simulink model "TST_OilT_VD"  (R2016b)
settings: Solver=FixedStepDiscrete  StartTime=0.0  StopTime=simTime  FixedStep=sampleTime  RelTol=1e-3
values from neighbouring files (symbols this model uses):
  testCase = 1    [initTST_OilT_VD_001.m]    (also in initTST_OilT_VD_002.m = 2)
libraries: UnitTest_Lib x8, simulink x3
settings Model: Creator=liangyunbo  LastModifiedBy=liangyunbo
settings DebuggingCC: SignalRangeChecking=error

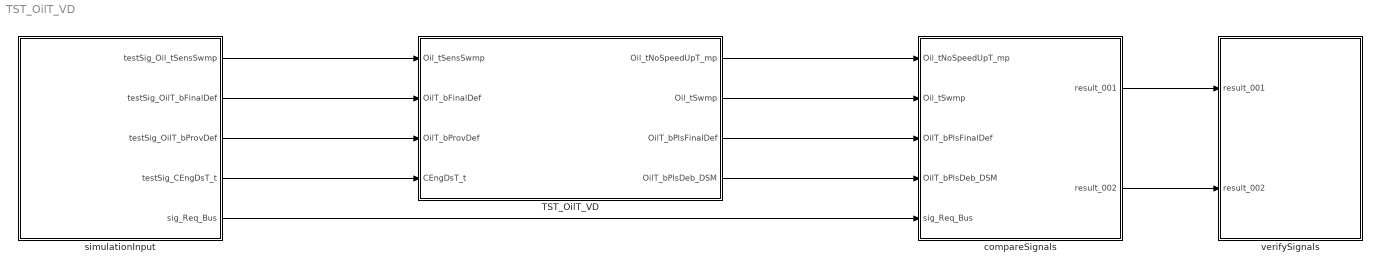
== system TST_OilT_VD ==
  TST_OilT_VD : Subsystem
  compareSignals : Subsystem
  simulationInput : Subsystem
  verifySignals : Subsystem
  wires:
  simulationInput/1(testSig_Oil_tSensSwmp) -> TST_OilT_VD/1(Oil_tSensSwmp)
  simulationInput/2(testSig_OilT_bFinalDef) -> TST_OilT_VD/2(OilT_bFinalDef)
  simulationInput/3(testSig_OilT_bProvDef) -> TST_OilT_VD/3(OilT_bProvDef)
  simulationInput/4(testSig_CEngDsT_t) -> TST_OilT_VD/4(CEngDsT_t)
  TST_OilT_VD/1(Oil_tNoSpeedUpT_mp) -> compareSignals/1(Oil_tNoSpeedUpT_mp)
  TST_OilT_VD/2(Oil_tSwmp) -> compareSignals/2(Oil_tSwmp)
  TST_OilT_VD/3(OilT_bPlsFinalDef) -> compareSignals/3(OilT_bPlsFinalDef)
  TST_OilT_VD/4(OilT_bPlsDeb_DSM) -> compareSignals/4(OilT_bPlsDeb_DSM)
  simulationInput/5(sig_Req_Bus) -> compareSignals/5(sig_Req_Bus)
  compareSignals/1(result_001) -> verifySignals/1(result_001)
  compareSignals/2(result_002) -> verifySignals/2(result_002)

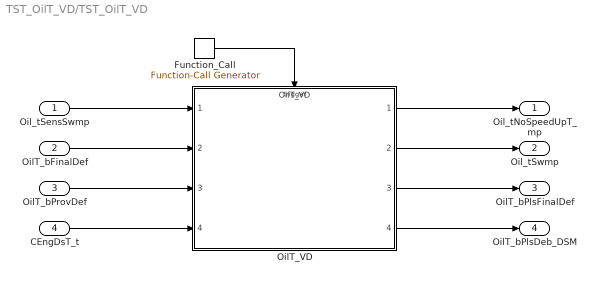
== system TST_OilT_VD/TST_OilT_VD ==
  Oil_tSensSwmp : Inport
  OilT_bFinalDef : Inport  Port=2
  OilT_bProvDef : Inport  Port=3
  CEngDsT_t : Inport  Port=4
  Function_Call : simulink/Ports & Subsystems/Function-Call Generator  sample_time=sampleTime  numberOfIterations=1
  OilT_VD : ModelReference  ModelNameDialog=OilT_VD  SimulationMode=Normal  ModelReferenceVersion=1.9  TriggerPortName=function  TriggerPortTriggerType=function-call  TriggerPortStatesWhenEnabling=held
  Oil_tNoSpeedUpT_mp : Outport
  Oil_tSwmp : Outport  Port=2
  OilT_bPlsFinalDef : Outport  Port=3
  OilT_bPlsDeb_DSM : Outport  Port=4
  wires:
  Function_Call/1 -> OilT_VD/Trigger
  Oil_tSensSwmp/1 -> OilT_VD/1
  OilT_bFinalDef/1 -> OilT_VD/2
  OilT_bProvDef/1 -> OilT_VD/3
  CEngDsT_t/1 -> OilT_VD/4
  OilT_VD/1 -> Oil_tNoSpeedUpT_mp/1
  OilT_VD/2 -> Oil_tSwmp/1
  OilT_VD/3 -> OilT_bPlsFinalDef/1
  OilT_VD/4 -> OilT_bPlsDeb_DSM/1

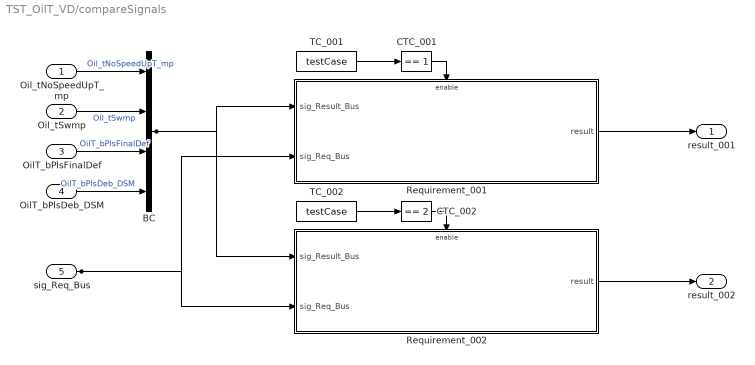
== system TST_OilT_VD/compareSignals ==
  Oil_tNoSpeedUpT_mp : Inport
  Oil_tSwmp : Inport  Port=2
  OilT_bPlsFinalDef : Inport  Port=3
  OilT_bPlsDeb_DSM : Inport  Port=4
  sig_Req_Bus : Inport  Port=5
  BC : BusCreator  Inputs=4
  CTC_001 : simulink/Logic and Bit Operations/Compare To Constant  relop===  const=1  OutDataTypeStr=boolean
  CTC_002 : simulink/Logic and Bit Operations/Compare To Constant  relop===  const=2  OutDataTypeStr=boolean
  Requirement_001 : Subsystem
  Requirement_002 : Subsystem
  TC_001 : Constant  Value=testCase
  TC_002 : Constant  Value=testCase
  result_001 : Outport
  result_002 : Outport  Port=2
  wires:
  Oil_tNoSpeedUpT_mp/1 -> BC/1  "Oil_tNoSpeedUpT_mp"
  Oil_tSwmp/1 -> BC/2  "Oil_tSwmp"
  OilT_bPlsFinalDef/1 -> BC/3  "OilT_bPlsFinalDef"
  OilT_bPlsDeb_DSM/1 -> BC/4  "OilT_bPlsDeb_DSM"
  TC_001/1 -> CTC_001/1
  CTC_001/1 -> Requirement_001/Enable
  sig_Req_Bus/1 -> Requirement_001/2(sig_Req_Bus), Requirement_002/2(sig_Req_Bus)
  BC/1 -> Requirement_001/1(sig_Result_Bus), Requirement_002/1(sig_Result_Bus)
  Requirement_001/1(result) -> result_001/1
  TC_002/1 -> CTC_002/1
  CTC_002/1 -> Requirement_002/Enable
  Requirement_002/1(result) -> result_002/1

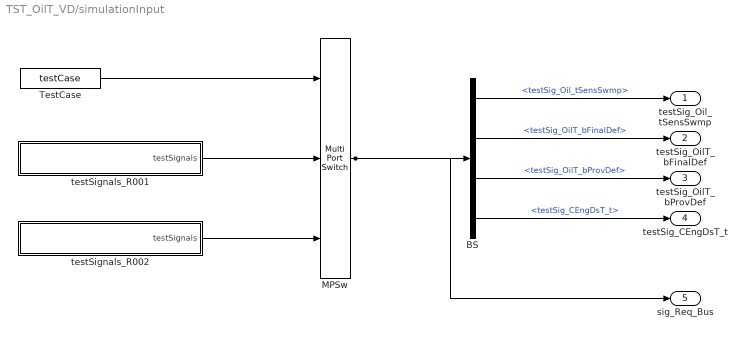
== system TST_OilT_VD/simulationInput ==
  BS : BusSelector  OutputSignals=testSig_Oil_tSensSwmp,testSig_OilT_bFinalDef,testSig_OilT_bProvDef,testSig_CEngDsT_t
  MPSw : MultiPortSwitch  Inputs=2  SaturateOnIntegerOverflow=on  InputSameDT=on
  TestCase : Constant  Value=testCase
  testSignals_R001 : Subsystem
  testSignals_R002 : Subsystem
  testSig_Oil_tSensSwmp : Outport
  testSig_OilT_bFinalDef : Outport  Port=2
  testSig_OilT_bProvDef : Outport  Port=3
  testSig_CEngDsT_t : Outport  Port=4
  sig_Req_Bus : Outport  Port=5
  wires:
  BS/1 -> testSig_Oil_tSensSwmp/1  "<testSig_Oil_tSensSwmp>"
  BS/2 -> testSig_OilT_bFinalDef/1  "<testSig_OilT_bFinalDef>"
  BS/3 -> testSig_OilT_bProvDef/1  "<testSig_OilT_bProvDef>"
  BS/4 -> testSig_CEngDsT_t/1  "<testSig_CEngDsT_t>"
  MPSw/1 -> BS/1, sig_Req_Bus/1
  TestCase/1 -> MPSw/1
  testSignals_R001/1(testSignals) -> MPSw/2
  testSignals_R002/1(testSignals) -> MPSw/3

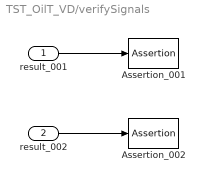
== system TST_OilT_VD/verifySignals ==
  result_001 : Inport
  result_002 : Inport  Port=2
  Assertion_001 : Assertion  Enabled=off
  Assertion_002 : Assertion  Enabled=off
  wires:
  result_001/1 -> Assertion_001/1
  result_002/1 -> Assertion_002/1

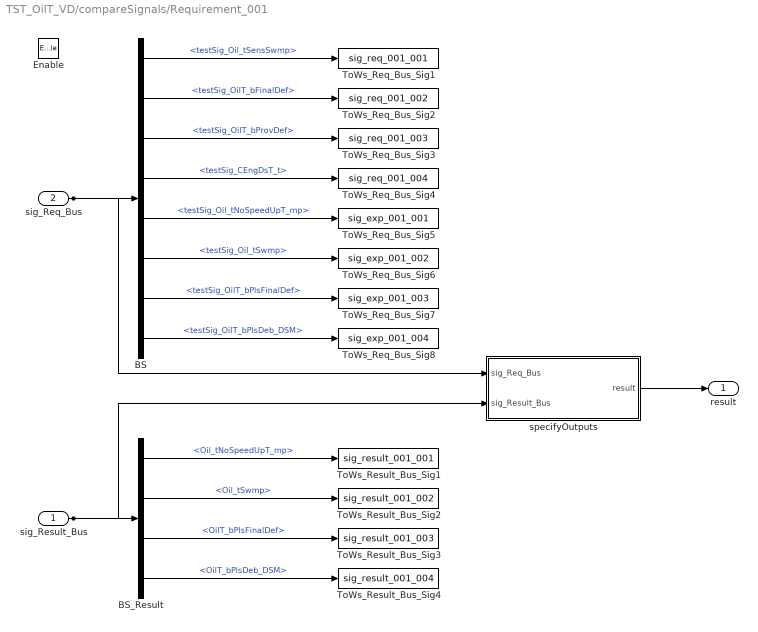
== system TST_OilT_VD/compareSignals/Requirement_001 ==
  sig_Result_Bus : Inport
  sig_Req_Bus : Inport  Port=2
  Enable : EnablePort
  BS : BusSelector  OutputSignals=testSig_Oil_tSensSwmp,testSig_OilT_bFinalDef,testSig_OilT_bProvDef,testSig_CEngDsT_t,testSig_Oil_tNoSpeedUpT_mp,testSig_Oil_tSwmp,testSig_OilT_bPlsFinalDef,testSig_OilT_bPlsDeb_DSM
  BS_Result : BusSelector  OutputSignals=Oil_tNoSpeedUpT_mp,Oil_tSwmp,OilT_bPlsFinalDef,OilT_bPlsDeb_DSM
  ToWs_Req_Bus_Sig1 : ToWorkspace  VariableName=sig_req_001_001  SaveFormat=Structure With Time
  ToWs_Req_Bus_Sig2 : ToWorkspace  VariableName=sig_req_001_002  SaveFormat=Structure With Time
  ToWs_Req_Bus_Sig3 : ToWorkspace  VariableName=sig_req_001_003  SaveFormat=Structure With Time
  ToWs_Req_Bus_Sig4 : ToWorkspace  VariableName=sig_req_001_004  SaveFormat=Structure With Time
  ToWs_Req_Bus_Sig5 : ToWorkspace  VariableName=sig_exp_001_001  SaveFormat=Structure With Time
  ToWs_Req_Bus_Sig6 : ToWorkspace  VariableName=sig_exp_001_002  SaveFormat=Structure With Time
  ToWs_Req_Bus_Sig7 : ToWorkspace  VariableName=sig_exp_001_003  SaveFormat=Structure With Time
  ToWs_Req_Bus_Sig8 : ToWorkspace  VariableName=sig_exp_001_004  SaveFormat=Structure With Time
  ToWs_Result_Bus_Sig1 : ToWorkspace  VariableName=sig_result_001_001  SaveFormat=Structure With Time
  ToWs_Result_Bus_Sig2 : ToWorkspace  VariableName=sig_result_001_002  SaveFormat=Structure With Time
  ToWs_Result_Bus_Sig3 : ToWorkspace  VariableName=sig_result_001_003  SaveFormat=Structure With Time
  ToWs_Result_Bus_Sig4 : ToWorkspace  VariableName=sig_result_001_004  SaveFormat=Structure With Time
  specifyOutputs : Subsystem
  result : Outport
  wires:
  sig_Req_Bus/1 -> BS/1, specifyOutputs/1(sig_Req_Bus)
  BS/1 -> ToWs_Req_Bus_Sig1/1  "<testSig_Oil_tSensSwmp>"
  BS/2 -> ToWs_Req_Bus_Sig2/1  "<testSig_OilT_bFinalDef>"
  BS/3 -> ToWs_Req_Bus_Sig3/1  "<testSig_OilT_bProvDef>"
  BS/4 -> ToWs_Req_Bus_Sig4/1  "<testSig_CEngDsT_t>"
  BS/5 -> ToWs_Req_Bus_Sig5/1  "<testSig_Oil_tNoSpeedUpT_mp>"
  BS/6 -> ToWs_Req_Bus_Sig6/1  "<testSig_Oil_tSwmp>"
  BS/7 -> ToWs_Req_Bus_Sig7/1  "<testSig_OilT_bPlsFinalDef>"
  BS/8 -> ToWs_Req_Bus_Sig8/1  "<testSig_OilT_bPlsDeb_DSM>"
  sig_Result_Bus/1 -> BS_Result/1, specifyOutputs/2(sig_Result_Bus)
  BS_Result/1 -> ToWs_Result_Bus_Sig1/1  "<Oil_tNoSpeedUpT_mp>"
  BS_Result/2 -> ToWs_Result_Bus_Sig2/1  "<Oil_tSwmp>"
  BS_Result/3 -> ToWs_Result_Bus_Sig3/1  "<OilT_bPlsFinalDef>"
  BS_Result/4 -> ToWs_Result_Bus_Sig4/1  "<OilT_bPlsDeb_DSM>"
  specifyOutputs/1(result) -> result/1

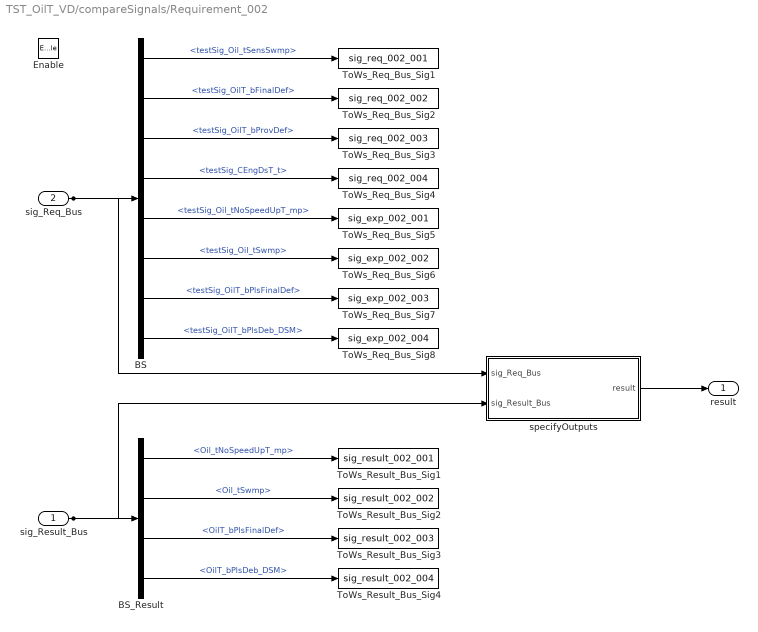
== system TST_OilT_VD/compareSignals/Requirement_002 ==
  sig_Result_Bus : Inport
  sig_Req_Bus : Inport  Port=2
  Enable : EnablePort
  BS : BusSelector  OutputSignals=testSig_Oil_tSensSwmp,testSig_OilT_bFinalDef,testSig_OilT_bProvDef,testSig_CEngDsT_t,testSig_Oil_tNoSpeedUpT_mp,testSig_Oil_tSwmp,testSig_OilT_bPlsFinalDef,testSig_OilT_bPlsDeb_DSM
  BS_Result : BusSelector  OutputSignals=Oil_tNoSpeedUpT_mp,Oil_tSwmp,OilT_bPlsFinalDef,OilT_bPlsDeb_DSM
  ToWs_Req_Bus_Sig1 : ToWorkspace  VariableName=sig_req_002_001  SaveFormat=Structure With Time
  ToWs_Req_Bus_Sig2 : ToWorkspace  VariableName=sig_req_002_002  SaveFormat=Structure With Time
  ToWs_Req_Bus_Sig3 : ToWorkspace  VariableName=sig_req_002_003  SaveFormat=Structure With Time
  ToWs_Req_Bus_Sig4 : ToWorkspace  VariableName=sig_req_002_004  SaveFormat=Structure With Time
  ToWs_Req_Bus_Sig5 : ToWorkspace  VariableName=sig_exp_002_001  SaveFormat=Structure With Time
  ToWs_Req_Bus_Sig6 : ToWorkspace  VariableName=sig_exp_002_002  SaveFormat=Structure With Time
  ToWs_Req_Bus_Sig7 : ToWorkspace  VariableName=sig_exp_002_003  SaveFormat=Structure With Time
  ToWs_Req_Bus_Sig8 : ToWorkspace  VariableName=sig_exp_002_004  SaveFormat=Structure With Time
  ToWs_Result_Bus_Sig1 : ToWorkspace  VariableName=sig_result_002_001  SaveFormat=Structure With Time
  ToWs_Result_Bus_Sig2 : ToWorkspace  VariableName=sig_result_002_002  SaveFormat=Structure With Time
  ToWs_Result_Bus_Sig3 : ToWorkspace  VariableName=sig_result_002_003  SaveFormat=Structure With Time
  ToWs_Result_Bus_Sig4 : ToWorkspace  VariableName=sig_result_002_004  SaveFormat=Structure With Time
  specifyOutputs : Subsystem
  result : Outport
  wires:
  sig_Req_Bus/1 -> BS/1, specifyOutputs/1(sig_Req_Bus)
  BS/1 -> ToWs_Req_Bus_Sig1/1  "<testSig_Oil_tSensSwmp>"
  BS/2 -> ToWs_Req_Bus_Sig2/1  "<testSig_OilT_bFinalDef>"
  BS/3 -> ToWs_Req_Bus_Sig3/1  "<testSig_OilT_bProvDef>"
  BS/4 -> ToWs_Req_Bus_Sig4/1  "<testSig_CEngDsT_t>"
  BS/5 -> ToWs_Req_Bus_Sig5/1  "<testSig_Oil_tNoSpeedUpT_mp>"
  BS/6 -> ToWs_Req_Bus_Sig6/1  "<testSig_Oil_tSwmp>"
  BS/7 -> ToWs_Req_Bus_Sig7/1  "<testSig_OilT_bPlsFinalDef>"
  BS/8 -> ToWs_Req_Bus_Sig8/1  "<testSig_OilT_bPlsDeb_DSM>"
  sig_Result_Bus/1 -> BS_Result/1, specifyOutputs/2(sig_Result_Bus)
  BS_Result/1 -> ToWs_Result_Bus_Sig1/1  "<Oil_tNoSpeedUpT_mp>"
  BS_Result/2 -> ToWs_Result_Bus_Sig2/1  "<Oil_tSwmp>"
  BS_Result/3 -> ToWs_Result_Bus_Sig3/1  "<OilT_bPlsFinalDef>"
  BS_Result/4 -> ToWs_Result_Bus_Sig4/1  "<OilT_bPlsDeb_DSM>"
  specifyOutputs/1(result) -> result/1

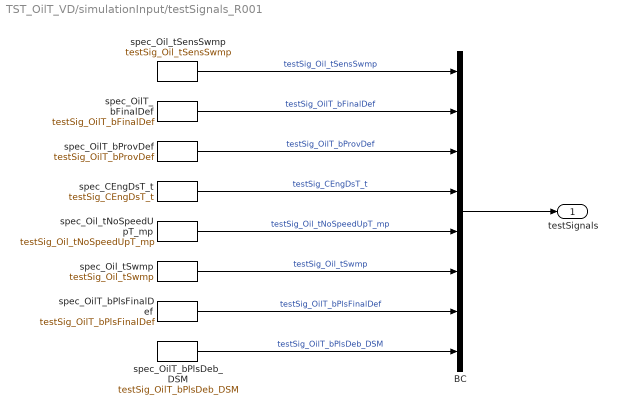
== system TST_OilT_VD/simulationInput/testSignals_R001 ==
  BC : BusCreator  Inputs=8
  spec_CEngDsT_t : FromWorkspace  VariableName=testSig_CEngDsT_t  Interpolate=off  OutputAfterFinalValue=Holding final value
  spec_OilT_bFinalDef : FromWorkspace  VariableName=testSig_OilT_bFinalDef  Interpolate=off  OutputAfterFinalValue=Holding final value
  spec_OilT_bPlsDeb_DSM : FromWorkspace  VariableName=testSig_OilT_bPlsDeb_DSM  Interpolate=off  OutputAfterFinalValue=Holding final value
  spec_OilT_bPlsFinalDef : FromWorkspace  VariableName=testSig_OilT_bPlsFinalDef  Interpolate=off  OutputAfterFinalValue=Holding final value
  spec_OilT_bProvDef : FromWorkspace  VariableName=testSig_OilT_bProvDef  Interpolate=off  OutputAfterFinalValue=Holding final value
  spec_Oil_tNoSpeedUpT_mp : FromWorkspace  VariableName=testSig_Oil_tNoSpeedUpT_mp  Interpolate=off  OutputAfterFinalValue=Holding final value
  spec_Oil_tSensSwmp : FromWorkspace  VariableName=testSig_Oil_tSensSwmp  Interpolate=off  OutputAfterFinalValue=Holding final value
  spec_Oil_tSwmp : FromWorkspace  VariableName=testSig_Oil_tSwmp  Interpolate=off  OutputAfterFinalValue=Holding final value
  testSignals : Outport
  wires:
  BC/1 -> testSignals/1
  spec_Oil_tSensSwmp/1 -> BC/1  "testSig_Oil_tSensSwmp"
  spec_OilT_bFinalDef/1 -> BC/2  "testSig_OilT_bFinalDef"
  spec_OilT_bProvDef/1 -> BC/3  "testSig_OilT_bProvDef"
  spec_CEngDsT_t/1 -> BC/4  "testSig_CEngDsT_t"
  spec_Oil_tNoSpeedUpT_mp/1 -> BC/5  "testSig_Oil_tNoSpeedUpT_mp"
  spec_Oil_tSwmp/1 -> BC/6  "testSig_Oil_tSwmp"
  spec_OilT_bPlsFinalDef/1 -> BC/7  "testSig_OilT_bPlsFinalDef"
  spec_OilT_bPlsDeb_DSM/1 -> BC/8  "testSig_OilT_bPlsDeb_DSM"

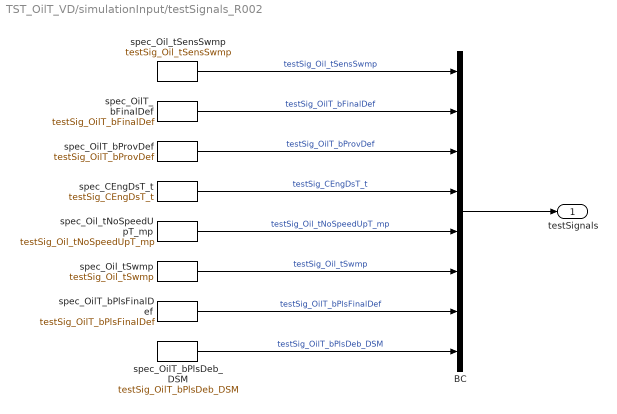
== system TST_OilT_VD/simulationInput/testSignals_R002 ==
  BC : BusCreator  Inputs=8
  spec_CEngDsT_t : FromWorkspace  VariableName=testSig_CEngDsT_t  Interpolate=off  OutputAfterFinalValue=Holding final value
  spec_OilT_bFinalDef : FromWorkspace  VariableName=testSig_OilT_bFinalDef  Interpolate=off  OutputAfterFinalValue=Holding final value
  spec_OilT_bPlsDeb_DSM : FromWorkspace  VariableName=testSig_OilT_bPlsDeb_DSM  Interpolate=off  OutputAfterFinalValue=Holding final value
  spec_OilT_bPlsFinalDef : FromWorkspace  VariableName=testSig_OilT_bPlsFinalDef  Interpolate=off  OutputAfterFinalValue=Holding final value
  spec_OilT_bProvDef : FromWorkspace  VariableName=testSig_OilT_bProvDef  Interpolate=off  OutputAfterFinalValue=Holding final value
  spec_Oil_tNoSpeedUpT_mp : FromWorkspace  VariableName=testSig_Oil_tNoSpeedUpT_mp  Interpolate=off  OutputAfterFinalValue=Holding final value
  spec_Oil_tSensSwmp : FromWorkspace  VariableName=testSig_Oil_tSensSwmp  Interpolate=off  OutputAfterFinalValue=Holding final value
  spec_Oil_tSwmp : FromWorkspace  VariableName=testSig_Oil_tSwmp  Interpolate=off  OutputAfterFinalValue=Holding final value
  testSignals : Outport
  wires:
  BC/1 -> testSignals/1
  spec_Oil_tSensSwmp/1 -> BC/1  "testSig_Oil_tSensSwmp"
  spec_OilT_bFinalDef/1 -> BC/2  "testSig_OilT_bFinalDef"
  spec_OilT_bProvDef/1 -> BC/3  "testSig_OilT_bProvDef"
  spec_CEngDsT_t/1 -> BC/4  "testSig_CEngDsT_t"
  spec_Oil_tNoSpeedUpT_mp/1 -> BC/5  "testSig_Oil_tNoSpeedUpT_mp"
  spec_Oil_tSwmp/1 -> BC/6  "testSig_Oil_tSwmp"
  spec_OilT_bPlsFinalDef/1 -> BC/7  "testSig_OilT_bPlsFinalDef"
  spec_OilT_bPlsDeb_DSM/1 -> BC/8  "testSig_OilT_bPlsDeb_DSM"

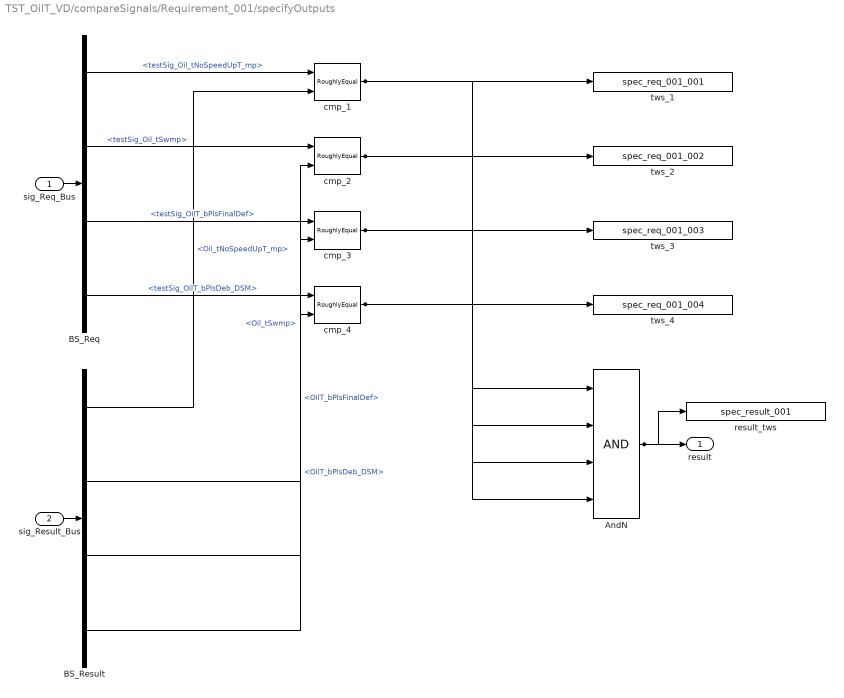
== system TST_OilT_VD/compareSignals/Requirement_001/specifyOutputs ==
  sig_Req_Bus : Inport
  sig_Result_Bus : Inport  Port=2
  AndN : Logic  Inputs=4
  BS_Req : BusSelector  OutputSignals=testSig_Oil_tNoSpeedUpT_mp,testSig_Oil_tSwmp,testSig_OilT_bPlsFinalDef,testSig_OilT_bPlsDeb_DSM
  BS_Result : BusSelector  OutputSignals=Oil_tNoSpeedUpT_mp,Oil_tSwmp,OilT_bPlsFinalDef,OilT_bPlsDeb_DSM
  cmp_{1..4} (4 alike) : UnitTest_Lib/RoughlyEqual  slope=0.1
  result_tws : ToWorkspace  VariableName=spec_result_001
  tws_1 : ToWorkspace  VariableName=spec_req_001_001
  tws_2 : ToWorkspace  VariableName=spec_req_001_002
  tws_3 : ToWorkspace  VariableName=spec_req_001_003
  tws_4 : ToWorkspace  VariableName=spec_req_001_004
  result : Outport
  wires:
  sig_Req_Bus/1 -> BS_Req/1
  sig_Result_Bus/1 -> BS_Result/1
  AndN/1 -> result/1, result_tws/1
  BS_Req/1 -> cmp_1/1  "<testSig_Oil_tNoSpeedUpT_mp>"
  BS_Result/1 -> cmp_1/2  "<Oil_tNoSpeedUpT_mp>"
  cmp_1/1 -> tws_1/1, AndN/1
  BS_Req/2 -> cmp_2/1  "<testSig_Oil_tSwmp>"
  BS_Result/2 -> cmp_2/2  "<Oil_tSwmp>"
  cmp_2/1 -> tws_2/1, AndN/2
  BS_Req/3 -> cmp_3/1  "<testSig_OilT_bPlsFinalDef>"
  BS_Result/3 -> cmp_3/2  "<OilT_bPlsFinalDef>"
  cmp_3/1 -> tws_3/1, AndN/3
  BS_Req/4 -> cmp_4/1  "<testSig_OilT_bPlsDeb_DSM>"
  BS_Result/4 -> cmp_4/2  "<OilT_bPlsDeb_DSM>"
  cmp_4/1 -> tws_4/1, AndN/4

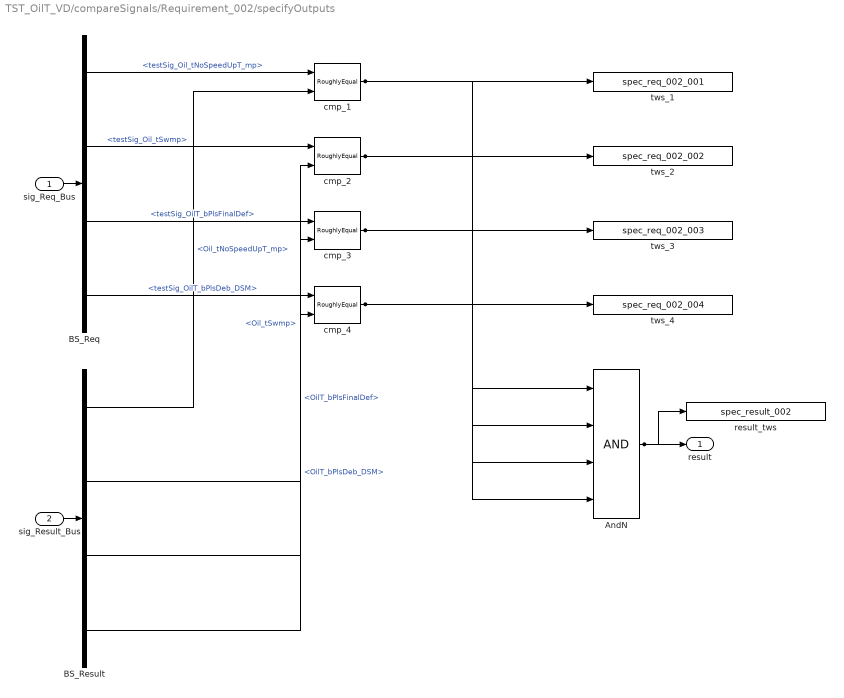
== system TST_OilT_VD/compareSignals/Requirement_002/specifyOutputs ==
  sig_Req_Bus : Inport
  sig_Result_Bus : Inport  Port=2
  AndN : Logic  Inputs=4
  BS_Req : BusSelector  OutputSignals=testSig_Oil_tNoSpeedUpT_mp,testSig_Oil_tSwmp,testSig_OilT_bPlsFinalDef,testSig_OilT_bPlsDeb_DSM
  BS_Result : BusSelector  OutputSignals=Oil_tNoSpeedUpT_mp,Oil_tSwmp,OilT_bPlsFinalDef,OilT_bPlsDeb_DSM
  cmp_{1..4} (4 alike) : UnitTest_Lib/RoughlyEqual  slope=0.1
  result_tws : ToWorkspace  VariableName=spec_result_002
  tws_1 : ToWorkspace  VariableName=spec_req_002_001
  tws_2 : ToWorkspace  VariableName=spec_req_002_002
  tws_3 : ToWorkspace  VariableName=spec_req_002_003
  tws_4 : ToWorkspace  VariableName=spec_req_002_004
  result : Outport
  wires:
  sig_Req_Bus/1 -> BS_Req/1
  sig_Result_Bus/1 -> BS_Result/1
  AndN/1 -> result/1, result_tws/1
  BS_Req/1 -> cmp_1/1  "<testSig_Oil_tNoSpeedUpT_mp>"
  BS_Result/1 -> cmp_1/2  "<Oil_tNoSpeedUpT_mp>"
  cmp_1/1 -> tws_1/1, AndN/1
  BS_Req/2 -> cmp_2/1  "<testSig_Oil_tSwmp>"
  BS_Result/2 -> cmp_2/2  "<Oil_tSwmp>"
  cmp_2/1 -> tws_2/1, AndN/2
  BS_Req/3 -> cmp_3/1  "<testSig_OilT_bPlsFinalDef>"
  BS_Result/3 -> cmp_3/2  "<OilT_bPlsFinalDef>"
  cmp_3/1 -> tws_3/1, AndN/3
  BS_Req/4 -> cmp_4/1  "<testSig_OilT_bPlsDeb_DSM>"
  BS_Result/4 -> cmp_4/2  "<OilT_bPlsDeb_DSM>"
  cmp_4/1 -> tws_4/1, AndN/4
